simulink model "PVFCHEV_1"  (R2018a)
settings: Solver=VariableStepAuto  StartTime=0.0  StopTime=25  RelTol=1e-3
values from neighbouring files (symbols this model uses):
  Fc_current = [ 0  1.7  3.3  5.06  6.8   8.6  10.4   12.3  14.15   16   17.85  19.8   21.8   23.75   25.75   27.75  29.8  31.9  34.1  36.2  38.2  40.9  42.6  44.7   47.1   49.4   51.6    54   56.85  58.75  61.2  63.6  66.1  68.6  71.2  73.8 76.5 79.15  81.85  84.6  87.5   90.4  93.3      96.4   99.45  102.5    105.65   109   112.8  115.75  119.25   123     126.65     130.5      134.5   138.6  142.9 147.4  153.0 ...(+15 chars)    [pvfchev_configration.m]
  Fc_power = [ 0  100  200  300   400   500   600    700   800   900   1000   1100   1200   1300    1400    1500  1600   1700  1800  1900  2000  2100  2200  2300   2400   2500   2600   2700   2800  2900   3000  3100  3200 3300   3400  3500 3600 3700  3800   3900   4000   4100  4198.5    4300   4400   4500      4600   4700  4800    4900    5000    5100     5200       5300       5400    5500  5600  5700   5800   ...(+17 chars)    [pvfchev_configration.m]
  Ts_Control = 1e-04    (= 0.0001)    [pvfchev_configration.m]
  Ts_Power = 2e-06    [pvfchev_configration.m]
undefined symbols (not defined in the file or in its folder): DiscIntNeverNeededParam, Ion, Lithium
libraries: powerlib x30, powerlib_meascontrol x8, sdl_lib x8, fl_lib x6, nesl_utility x6, electricdrivelib x4, spsVIMeasurementModel x3, simulink x2, re_lib x1, spsDrivesPrivateModels x1, spsDrivesOutputSelector x1, spsDrivesSpeedControllerModel x1
(part 2 of 2)

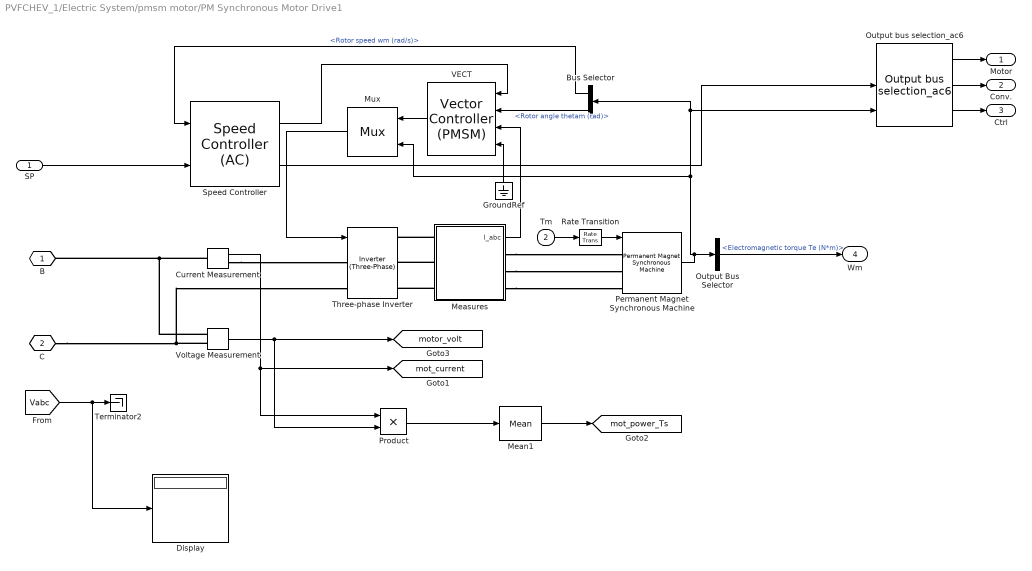
== system PVFCHEV_1/Electric System/pmsm motor/PM Synchronous Motor Drive1 ==
  SP : Inport
  Tm : Inport  Port=2
  Bus Selector : BusSelector  OutputSignals=Rotor speed wm (rad/s),Rotor angle thetam (rad)
  Current Measurement : powerlib/Measurements/Current Measurement  PhasorSimulation=off  OutputType=Complex  PSBequivalent=0
  Display : Display
  GroundRef : Ground
  Mean1 : powerlib_meascontrol/Measurements/Mean  Freq=60  Vinit=0  Ts=Ts_Control
  Measures : Subsystem
  Mux : spsDrivesPrivateModels/Mux  OverrideUsingVariant=Detailed  detailLevel=Detailed  driveType=AC6
      settings: AttributesFormatString=%<BlockChoice>  SourceProductName=The database C:\Users\ak23510\AppData\Roaming\MathWorks\MATLAB\R2017a\slblocks_master.db is locked, or a table in the database is locked. (database is locked)
  Output Bus Selector : BusSelector  OutputSignals=Electromagnetic torque Te (N*m)
  Output bus selection_ac6 : spsDrivesOutputSelector/Output bus selection_ac6  OverrideUsingVariant=Multiple_output_buses
      settings: AttributesFormatString=%<BlockChoice>  SourceProductName=The database C:\Users\ak23510\AppData\Roaming\MathWorks\MATLAB\R2017a\slblocks_master.db is locked, or a table in the database is locked. (database is locked)
  Permanent Magnet Synchronous Machine : powerlib/Machines/Permanent Magnet Synchronous Machine  NbPhases=3  FluxDistribution=Sinusoidal  RotorType=Salient-pole  MechanicalLoad=Speed w  PresetModel=No  ShowDetailedParameters=on  MeasurementBus=off  Resistance=Rs  Inductance=0  dqInductances=[Lls,Lms]  La=0.000835  MachineConstant=Flux linkage established by magnets (V.s)  Flux=0.28  VoltageCst=50.7864  TorqueCst=0.42  Flat=0  Mechanical=[J,Friction,p]  PolePairs=1  InitialConditions=[wm,thetam,ia,ib]  InitialConditions5ph=[0 0 0 0 0 0]  TsPowergui=0  TsBlock=-1  RefAngle=90 degrees behind phase A axis (modified Park)
      settings: AttributesFormatString=\n  SourceProductName=Simscape Power Systems
  Product : Product
  Rate Transition : RateTransition  OutPortSampleTime=baseSampleTime
  Speed Controller : spsDrivesSpeedControllerModel/Speed Controller (AC)  OverrideUsingVariant=AC345  ctrlType=Without flux reference output  SwK=Torque regulation  Ts=baseSampleTime  ramp=[Dec,Acc]  kp=kp_sc  ki=ki_sc  fc=fc_sc  ctrl_sat=[-120,50]  Tsc=Tsc  fn=60  p=2  nf=0.3
      settings: SourceProductName=The database C:\Users\ak23510\AppData\Roaming\MathWorks\MATLAB\R2017a\slblocks_master.db is locked, or a table in the database is locked. (database is locked)
  Terminator2 : Terminator
  Three-phase Inverter : electricdrivelib/Fundamental Drive Blocks/Inverter (Three-Phase)  OverrideUsingVariant=Detailed  detailLevel=Detailed  driveType=PMSM vector control  Ts=baseSampleTime  SnubberResistance=Rsnb_inv  SnubberCapacitance=Csnb_inv  Device=IGBT / Diodes  Ron=Ron_inv  ForwardVoltages="[  Vf_inv  Vfd_inv  ]"  GTOparameters=[Tf_GTO,Tt_GTO]  IGBTparameters="[  Tf  Tt  ]"  Measurements=All voltages and currents  converterType=Inverter  SourceFrequency=sourceFrequency  ReferenceFrame=Rotor  dqInductances=[Lls,Lms]  Inductance=0  Ls=0  Resistance=Rs  Flux=FluxCst  Stator_sm=[2.01e-3,4.289e-4,4.477e-3,1.354e-3]  Stator_im=[14.85e-3,0.3027e-3]  Rotor=[9.295e-3,0.3027e-3]  Lm=10.46e-3  p=p
      settings: AttributesFormatString=%<BlockChoice>  SourceProductName=Simscape Power Systems  SourceProductBaseCode=PS
  VECT : electricdrivelib/Fundamental Drive Blocks/Vector Controller (PMSM)  OverrideUsingVariant=Detailed_3ph  detailLevel=Detailed  nb_ph=3  modulationType=Hysteresis  Ts_vect=Tvect  h=h  freq_max=freq_max  fc_bus=fc_bus  car_freq=car_freq  nb_p=p  machineConstant=Flux linkage established by magnets (V.s)  fluxConstant=FluxCst  voltageConstant=VoltageCst  torqueConstant=TorqueCst  kp_Id=kp_Id  ki_Id=ki_Id  kp_Iq=kp_Iq  ki_Iq=ki_Iq
      settings: AttributesFormatString=%<BlockChoice>  SourceProductName=Simscape Power Systems  SourceProductBaseCode=PS
  Voltage Measurement : powerlib/Measurements/Voltage Measurement  PhasorSimulation=off  OutputType=Complex  PSBequivalent=0
  B : PMIOPort  Side=Left
  C : PMIOPort  Tag=PMCPort  Port=2  Side=Left
  Motor : Outport
  Conv. : Outport  Port=2
  Ctrl : Outport  Port=3
  Wm : Outport  Port=4
  tag scope: mot_current=global, mot_power_Ts=global, motor_volt=global
  wires:
  GroundRef/1 -> VECT/4
  Bus Selector/2 -> VECT/2  "<Rotor angle thetam (rad)>"
  Bus Selector/1 -> Speed Controller/1  "<Rotor speed wm (rad/s)>"
  VECT/1 -> Mux/1
  Speed Controller/2 -> Output bus selection_ac6/2
  Measures/1(I_abc) -> VECT/3
  Permanent Magnet Synchronous Machine/1 -> Bus Selector/1, Output bus selection_ac6/3, Mux/2, Output Bus Selector/1
  SP/1 -> Speed Controller/2
  Output Bus Selector/1 -> Wm/1  "<Electromagnetic torque Te (N*m)>"
  Rate Transition/1 -> Permanent Magnet Synchronous Machine/1
  Output bus selection_ac6/2 -> Conv./1
  Output bus selection_ac6/3 -> Ctrl/1
  Output bus selection_ac6/1 -> Motor/1
  Speed Controller/1 -> VECT/1
  Mux/1 -> Three-phase Inverter/1
  Tm/1 -> Rate Transition/1
  [Vabc] -> Display/1, Terminator2/1
  Current Measurement/1 -> [mot_current], Product/1
  Voltage Measurement/1 -> [motor_volt], Product/2
  Product/1 -> Mean1/1
  Mean1/1 -> [mot_power_Ts]
  connections:
  Measures/LConn3 -- Three-phase Inverter/RConn3
  Measures/LConn2 -- Three-phase Inverter/RConn2
  Measures/LConn1 -- Three-phase Inverter/RConn1
  Measures/RConn3 -- Permanent Magnet Synchronous Machine/LConn3
  Measures/RConn2 -- Permanent Magnet Synchronous Machine/LConn2
  Measures/RConn1 -- Permanent Magnet Synchronous Machine/LConn1
  C/RConn1 -- Three-phase Inverter/LConn2 -- Voltage Measurement/LConn2
  Current Measurement/LConn1 -- B/RConn1 -- Voltage Measurement/LConn1
  Current Measurement/RConn1 -- Three-phase Inverter/LConn1

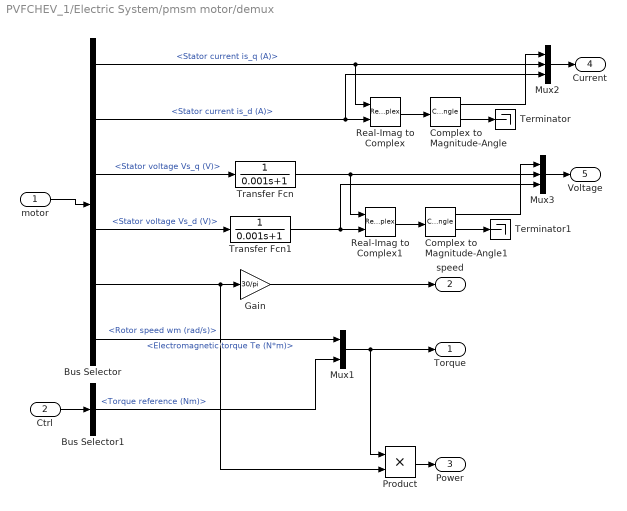
== system PVFCHEV_1/Electric System/pmsm motor/demux ==
  motor : Inport
  Ctrl : Inport  Port=2
  Bus Selector : BusSelector  OutputSignals=Stator current is_q (A),Stator current is_d (A),Stator voltage Vs_q (V),Stator voltage Vs_d (V),Rotor speed wm (rad/s),Electromagnetic torque Te (N*m)
  Bus Selector1 : BusSelector  OutputSignals=Torque reference (Nm)
  Complex to Magnitude-Angle : ComplexToMagnitudeAngle
  Complex to Magnitude-Angle1 : ComplexToMagnitudeAngle
  Gain : Gain  Gain=30/pi  SaturateOnIntegerOverflow=on  OutDataTypeStr=Inherit: Same as input  ParamDataTypeStr=Inherit: Same as input
  Mux1 : Mux  Inputs=2
  Mux2 : Mux  Inputs=3
  Mux3 : Mux  Inputs=3
  Product : Product  RndMeth=Zero
  Real-Imag to Complex : RealImagToComplex
  Real-Imag to Complex1 : RealImagToComplex
  Terminator : Terminator
  Terminator1 : Terminator
  Transfer Fcn : TransferFcn  Denominator=[0.001 1]
  Transfer Fcn1 : TransferFcn  Denominator=[0.001 1]
  Torque : Outport
  speed : Outport  Port=2
  Power : Outport  Port=3
  Current : Outport  Port=4
  Voltage : Outport  Port=5
  wires:
  Bus Selector/5 -> Gain/1, Product/2  "<Rotor speed wm (rad/s)>"
  Ctrl/1 -> Bus Selector1/1
  Gain/1 -> speed/1
  Mux1/1 -> Torque/1, Product/1
  motor/1 -> Bus Selector/1
  Mux2/1 -> Current/1
  Product/1 -> Power/1
  Bus Selector/2 -> Real-Imag to Complex/2, Mux2/3  "<Stator current is_d (A)>"
  Bus Selector/1 -> Real-Imag to Complex/1, Mux2/2  "<Stator current is_q (A)>"
  Real-Imag to Complex/1 -> Complex to Magnitude-Angle/1
  Complex to Magnitude-Angle/2 -> Terminator/1
  Complex to Magnitude-Angle/1 -> Mux2/1
  Mux3/1 -> Voltage/1
  Bus Selector/4 -> Transfer Fcn1/1  "<Stator voltage Vs_d (V)>"
  Bus Selector/3 -> Transfer Fcn/1  "<Stator voltage Vs_q (V)>"
  Real-Imag to Complex1/1 -> Complex to Magnitude-Angle1/1
  Complex to Magnitude-Angle1/2 -> Terminator1/1
  Complex to Magnitude-Angle1/1 -> Mux3/1
  Transfer Fcn/1 -> Mux3/2, Real-Imag to Complex1/1
  Transfer Fcn1/1 -> Mux3/3, Real-Imag to Complex1/2
  Bus Selector/6 -> Mux1/1  "<Electromagnetic torque Te (N*m)>"
  Bus Selector1/1 -> Mux1/2  "<Torque reference (Nm)>"

== system PVFCHEV_1/Electric System/mppt converter/Boost Converter (Average Model)/Prediction ==
  In : Inport
  Gain : Gain  Gain=2
  Subtract2 : Sum  Inputs=+-
  prediction : UnitDelay  SampleTime=Ts
  Out : Outport
  wires:
  prediction/1 -> Subtract2/2
  In/1 -> prediction/1, Gain/1
  Subtract2/1 -> Out/1
  Gain/1 -> Subtract2/1

== system PVFCHEV_1/Electric System/mppt converter/Boost Converter (Average Model)/scaling1 ==
  note: Shifting from ]0 to 1[ to a ]-1 to 1[ scale
  D : Inport
  Bias : Bias  Bias=-0.5
  Gain : Gain  Gain=2
  Saturation : Saturate  UpperLimit=1  LowerLimit=-1
  m : Outport
  wires:
  Saturation/1 -> m/1
  Gain/1 -> Saturation/1
  D/1 -> Bias/1
  Bias/1 -> Gain/1

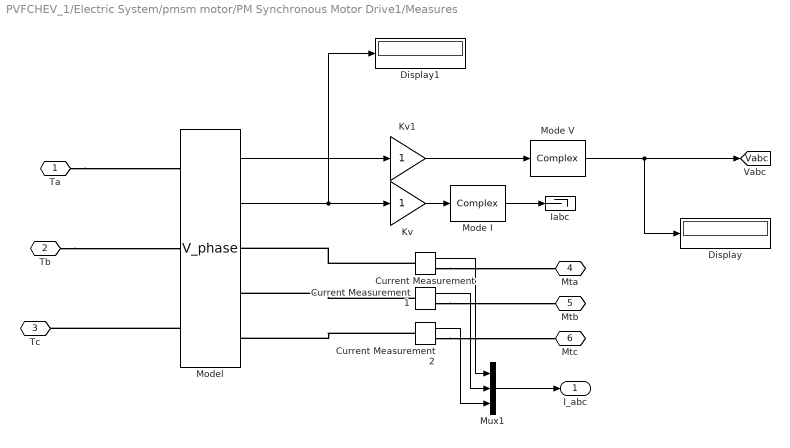
== system PVFCHEV_1/Electric System/pmsm motor/PM Synchronous Motor Drive1/Measures ==
  Current Measurement : powerlib/Measurements/Current Measurement  Tag=PoWeRsYsTeMmEaSuReMeNt  PhasorSimulation=off  OutputType=Magnitude  PSBequivalent=0
  Current Measurement1 : powerlib/Measurements/Current Measurement  Tag=PoWeRsYsTeMmEaSuReMeNt  PhasorSimulation=off  OutputType=Magnitude  PSBequivalent=0
  Current Measurement2 : powerlib/Measurements/Current Measurement  Tag=PoWeRsYsTeMmEaSuReMeNt  PhasorSimulation=off  OutputType=Magnitude  PSBequivalent=0
  Display : Display
  Display1 : Display
  Iabc : Terminator
  Kv : Gain  SaturateOnIntegerOverflow=on  OutDataTypeStr=Inherit: Same as input  ParamDataTypeStr=Inherit: Same as input
  Kv1 : Gain  SaturateOnIntegerOverflow=on  OutDataTypeStr=Inherit: Same as input  ParamDataTypeStr=Inherit: Same as input
  Mode I : spsVIMeasurementModel/Complex
  Mode V : spsVIMeasurementModel/Complex
  Model : spsVIMeasurementModel/V_phase  SystemSampleTime=-1
  Mux1 : Mux  Inputs=3
  Ta : PMIOPort  Side=Left
  Tb : PMIOPort  Port=2  Side=Left
  Tc : PMIOPort  Port=3  Side=Left
  Mta : PMIOPort  Port=4  Side=Right
  Mtb : PMIOPort  Port=5  Side=Right
  Mtc : PMIOPort  Port=6  Side=Right
  I_abc : Outport
  tag scope: Vabc=global
  wires:
  Mux1/1 -> I_abc/1
  Current Measurement2/1 -> Mux1/3
  Current Measurement/1 -> Mux1/1
  Current Measurement1/1 -> Mux1/2
  Mode V/1 -> Display/1, [Vabc]
  Kv1/1 -> Mode V/1
  Mode I/1 -> Iabc/1
  Kv/1 -> Mode I/1
  Model/2 -> Display1/1, Kv/1
  Model/1 -> Kv1/1
  connections:
  Current Measurement2/RConn1 -- Mtc/RConn1
  Current Measurement/RConn1 -- Mta/RConn1
  Current Measurement1/RConn1 -- Mtb/RConn1
  Tb/RConn1 -- Model/LConn2
  Current Measurement2/LConn1 -- Model/RConn3
  Ta/RConn1 -- Model/LConn1
  Current Measurement1/LConn1 -- Model/RConn2
  Model/LConn3 -- Tc/RConn1
  Current Measurement/LConn1 -- Model/RConn1

== matlab function PVFCHEV_1/Electric System/mppt converter/MPPT Controller using Perturbe & Observe technique  ==
  settings: updateMethod=DISCRETE  sampleTime=Ts_Control
  data: Param input; Enabled input; V input =V; I input; D output
function D  = PandO(Param, Enabled, V, I)

% MPPT controller based on the Perturb & Observe algorithm.

% D output = Duty cycle of the boost converter (value between 0 and 1)
%
% Enabled input = 1 to enable the MPPT controller
% V input = PV array terminal voltage (V)
% I input = PV array current (A)
%
% Param input:
Dinit = Param(1);  %Initial value for D output
Dmax = Param(2);   %Maximum value for D
Dmin = Param(3);   %Minimum value for D
deltaD = Param(4); %Increment value used to increase/decrease the duty cycle D
% ( increasing D = decreasing Vref )
%  

persistent Vold Pold Dold;

dataType = 'double';

if isempty(Vold)
    Vold=0;
    Pold=0;
    Dold=Dinit;
end
P= V*I;
dV= V - Vold;
dP= P - Pold;

if dP ~= 0 & Enabled ~=0
    if dP < 0
        if dV < 0
            D = Dold - deltaD;
        else
            D = Dold + deltaD;
        end
    else
        if dV < 0
            D = Dold + deltaD;
        else
            D = Dold - deltaD;
        end    
    end
else D=Dold;
end

if D >= Dmax | D<= Dmin
    D=Dold;
end

Dold=D;
Vold=V;
Pold=P;
